simulink model "Filter"  (R2020b)
settings: Solver=VariableStepAuto  StartTime=0.0  StopTime=100.0  RelTol=1e-3
settings Model: Creator=smart  LastModifiedBy=smart

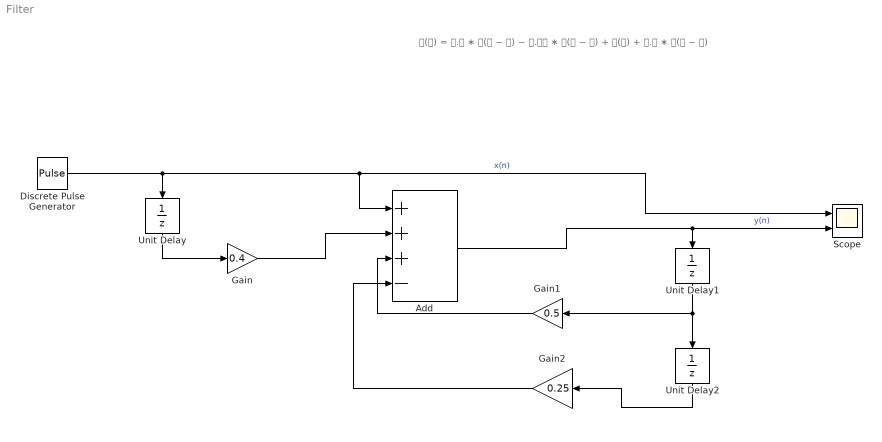
== system Filter ==
  note: 𝐲(𝐧) = 𝟎.𝟓 ∗ 𝐲(𝐧 − 𝟏) − 𝟎.𝟐𝟓 ∗ 𝐲(𝐧 − 𝟐) + 𝐱(𝐧) + 𝟎.𝟒 ∗ 𝐱(𝐧 − 𝟏)
  Add : Sum  Inputs=+++-
  Discrete Pulse Generator : DiscretePulseGenerator  Period=10
  Gain : Gain  Gain=0.4
  Gain1 : Gain  Gain=0.5
  Gain2 : Gain  Gain=0.25
  Scope : Scope  NumInputPorts=2
  Unit Delay : UnitDelay  SampleTime=-1  HasFrameUpgradeWarning=on
  Unit Delay1 : UnitDelay  SampleTime=-1  HasFrameUpgradeWarning=on
  Unit Delay2 : UnitDelay  SampleTime=-1  HasFrameUpgradeWarning=on
  wires:
  Gain/1 -> Add/2
  Unit Delay/1 -> Gain/1
  Discrete Pulse Generator/1 -> Scope/1, Add/1, Unit Delay/1  "x(n)"
  Add/1 -> Scope/2, Unit Delay1/1  "y(n)"
  Unit Delay1/1 -> Gain1/1, Unit Delay2/1
  Gain1/1 -> Add/3
  Gain2/1 -> Add/4
  Unit Delay2/1 -> Gain2/1
